simulink model "calculator"  (R2021b)
settings: Solver=VariableStepAuto  StartTime=0.0  StopTime=10.0  RelTol=1e-3
settings Model: Creator=midol  LastModifiedBy=midol

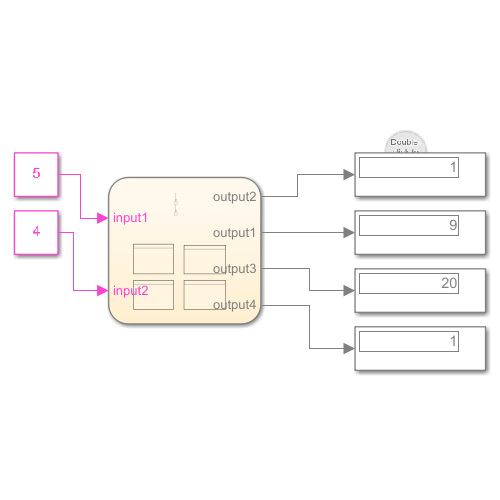
[thumbnail: Simulink's stored preview of the top-level diagram]
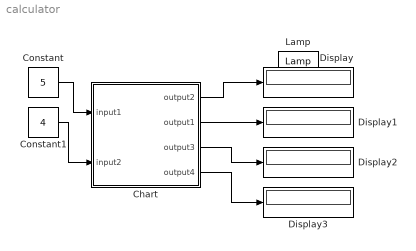
== system calculator ==
  Chart : Stateflow chart  TreatAsAtomicUnit=on
  Constant : Constant  Value=5
  Constant1 : Constant  Value=4
  Display{,1..3} (4 alike) : Display
  Lamp : LampBlock  LabelPosition=Hide
  wires:
  Constant/1 -> Chart/1(input1)
  Constant1/1 -> Chart/2(input2)
  Chart/1(output2) -> Display/1
  Chart/2(output1) -> Display1/1
  Chart/3(output3) -> Display2/1
  Chart/4(output4) -> Display3/1

== stateflow chart calculator/Chart ==
  state j=addation(x,y) [function]
    (default) -> (junction 21) : {j=x+y;}
  state m=subtraction(a,b) [function]
    (default) -> (junction 24) : {m=a-b;}
  state k=multiplication(x,y) [function]
    (default) -> (junction 37) : {k=x*y;}
  state f=division(x,y) [function]
    (default) -> (junction 40) : {f=x-y;}
  (default) -> (junction 26)
  (junction 26) -> (junction 28) : {
      | output1=addation(input1, input2);
      | output2 = subtraction(input1, input2);
      | output3 = multiplication(input1,input2);
      | output4 = division(input1, input2);
      |  }
  data: x function_input; y function_input; j function_output; a function_input; b function_input; m function_output; x function_input; y function_input; k function_output; x function_input; y function_input; f function_output; output2 output; output1 output; input1 input; input2 input; output3 output; output4 output
